simulink model "simple_quadcopter"  (R2019b)
settings: Solver=VariableStepAuto  StartTime=0.0  StopTime=10.0  RelTol=1e-3
values from neighbouring files (symbols this model uses):
  b = 3.0 *10^-5    (= 3e-05)    [constants_drone.m]    (also in drone.m)
  d = 1.1*10^-6    (= 1.1e-06)    [constants_drone.m]    (also in drone.m)
  Ixx = 6.12*10^-2    (= 0.0612)    [constants_drone.m]
  Iyy = Ixx    (= 0.0612)    [constants_drone.m]
  Izz = 8.11*10^-2    (= 0.0811)    [constants_drone.m]
  l = 0.225    [constants_drone.m]    (also in drone.m = 0.25)
  omega1 = 220    [constants_drone.m]
  omega2 = 219    [constants_drone.m]
  omega3 = 220    [constants_drone.m]
  omega4 = 220    [constants_drone.m]
settings Model: Creator=Emil  LastModifiedBy=Emil

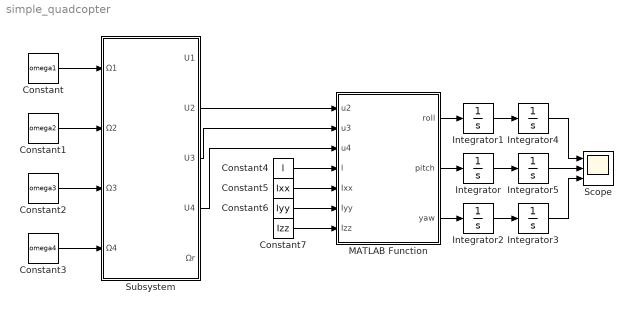
== system simple_quadcopter ==
  Constant : Constant  Value=omega1
  Constant1 : Constant  Value=omega2
  Constant2 : Constant  Value=omega3
  Constant3 : Constant  Value=omega4
  Constant4 : Constant  Value=l
  Constant5 : Constant  Value=Ixx
  Constant6 : Constant  Value=Iyy
  Constant7 : Constant  Value=Izz
  Integrator{,1..5} (6 alike) : Integrator
  MATLAB Function : MATLAB Function  TreatAsAtomicUnit=on
  Scope : Scope  NumInputPorts=3
  Subsystem : Subsystem
  wires:
  Constant/1 -> Subsystem/1(Ω1)
  Constant1/1 -> Subsystem/2(Ω2)
  Constant2/1 -> Subsystem/3(Ω3)
  Constant3/1 -> Subsystem/4(Ω4)
  Subsystem/2(U2) -> MATLAB Function/1(u2)
  Subsystem/3(U3) -> MATLAB Function/2(u3)
  Subsystem/4(U4) -> MATLAB Function/3(u4)
  Constant4/1 -> MATLAB Function/4(l)
  Constant5/1 -> MATLAB Function/5(Ixx)
  Constant6/1 -> MATLAB Function/6(Iyy)
  MATLAB Function/2(pitch) -> Integrator/1
  MATLAB Function/1(roll) -> Integrator1/1
  MATLAB Function/3(yaw) -> Integrator2/1
  Constant7/1 -> MATLAB Function/7(Izz)
  Integrator1/1 -> Integrator4/1
  Integrator/1 -> Integrator5/1
  Integrator2/1 -> Integrator3/1
  Integrator3/1 -> Scope/3
  Integrator4/1 -> Scope/1
  Integrator5/1 -> Scope/2

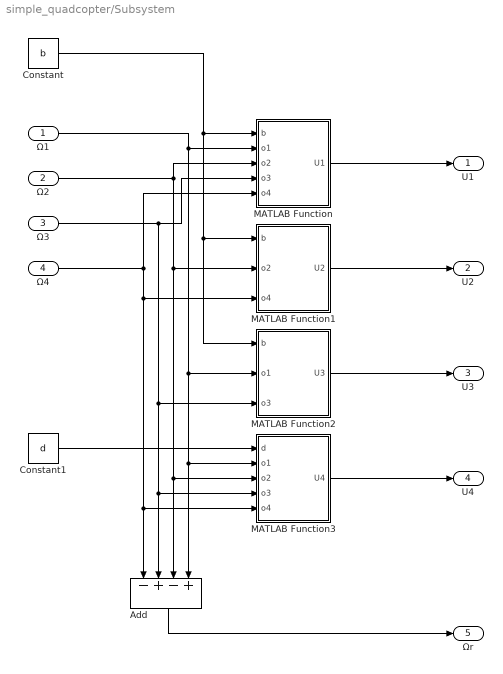
== system simple_quadcopter/Subsystem ==
  Ω1 : Inport
  Ω2 : Inport  Port=2
  Ω3 : Inport  Port=3
  Ω4 : Inport  Port=4
  Add : Sum  Inputs=-+-+
  Constant : Constant  Value=b
  Constant1 : Constant  Value=d
  MATLAB Function : MATLAB Function  TreatAsAtomicUnit=on
  MATLAB Function1 : MATLAB Function  TreatAsAtomicUnit=on
  MATLAB Function2 : MATLAB Function  TreatAsAtomicUnit=on
  MATLAB Function3 : MATLAB Function  TreatAsAtomicUnit=on
  U1 : Outport
  U2 : Outport  Port=2
  U3 : Outport  Port=3
  U4 : Outport  Port=4
  Ωr : Outport  Port=5
  wires:
  Add/1 -> Ωr/1
  Ω4/1 -> MATLAB Function1/3(o4), MATLAB Function3/5(o4), Add/1, MATLAB Function/5(o4)
  Ω3/1 -> MATLAB Function2/3(o3), MATLAB Function3/4(o3), Add/2, MATLAB Function/4(o3)
  Ω2/1 -> MATLAB Function/3(o2), MATLAB Function1/2(o2), MATLAB Function3/3(o2), Add/3
  Ω1/1 -> MATLAB Function2/2(o1), MATLAB Function3/2(o1), Add/4, MATLAB Function/2(o1)
  MATLAB Function/1(U1) -> U1/1
  MATLAB Function1/1(U2) -> U2/1
  MATLAB Function2/1(U3) -> U3/1
  MATLAB Function3/1(U4) -> U4/1
  Constant/1 -> MATLAB Function2/1(b), MATLAB Function1/1(b), MATLAB Function/1(b)
  Constant1/1 -> MATLAB Function3/1(d)

== matlab function simple_quadcopter/Subsystem/MATLAB Function1 ==
  data: b input; U2 output; o2 input; o4 input
function U2 = fcn(b, o2, o4)

U2 = b*(-o2^2+o4^2);

== matlab function simple_quadcopter/Subsystem/MATLAB Function ==
  data: b input; U1 output; o1 input; o2 input; o3 input; o4 input
function U1 = fcn(b, o1, o2, o3, o4)

U1 = b*(o1^2+o2^2+o3^2+o4^2);

== matlab function simple_quadcopter/Subsystem/MATLAB Function2 ==
  data: b input; U3 output; o1 input; o3 input
function U3 = fcn(b, o1, o3)

U3 = b*(o1^2-o3^2);

== matlab function simple_quadcopter/Subsystem/MATLAB Function3 ==
  data: d input; U4 output; o1 input; o2 input; o3 input; o4 input
function U4 = fcn(d, o1, o2, o3, o4)

U4 = d*(o1^2-o2^2+o3^2-o4^2);

== matlab function simple_quadcopter/MATLAB Function ==
  data: u2 input; roll output; u3 input; u4 input; pitch output; yaw output; l input; Ixx input; Iyy input; Izz input
function [roll,pitch,yaw]= fcn(u2, u3, u4, l, Ixx, Iyy, Izz)

roll = l*(u2/Ixx);
pitch = l*(u3/Iyy);
yaw = l*(u4/Izz);
